simulink model "cartpole_baseline"  (R2026a)
settings: Solver=VariableStepAuto  StopTime=120
InitFcn:
  | cartpole_system_init
undefined symbols (not defined in the file): A, B_u, C, K, L, p, X, x0_i, x0_phys, Y, Z
libraries: sm_lib x9, nesl_utility x3
settings Model: Creator=david  LastModifiedBy=david
settings ExplorerConfigSet: InternalSimMechanicsExplorerSettings=|
  | <ExplorerConfiguration>
  | 
  |   <canonicalview>default</canonicalview>
  | 
  |   <TilePanel>
  |     <TileInfo>
  |       <Tiles Columns="1" Count="1" Height="610" Rows="1" Width="1536">
  |         <Row Weight="1"/>
  |         <Column Weight="1"/>
  |         <Tile Height="1" Width="1" X="0" Y="0"/>
  |       </Tiles>
  |     </TileInfo>
  |     <SceneInfo>
  |       <SceneViewer>
  |         <IsThisViewStd>
  |           <IsStandardView>off</IsStandardView>
  |           <StandardViewName>Front</StandardViewName>
  |         </IsThisViewStd>
  |         <BGColor>
  |           <R>1</R>
  |           <G>1</G>
  |           <B>1</B>
  |           <A>1</A>
  |         </BGColor>
  |         <Camera>
  |           <DoPerspective>off</DoPerspective>
  |           <Position>
  |             <X>-0.38733030516761002</X>
  |             <Y>0.60926147831297028</Y>
  |             <Z>3.3549500429517707</Z>
  |           </Position>
  |           <Center>
  |             <X>-0.38733030516761002</X>
  |             <Y>0.60926147831297028</Y>
  |             <Z>-0.019999999403953556</Z>
  |           </Center>
  |           <Up>
  |             <X>0</X>
  |             <Y>1</Y>
  |             <Z>0</Z>
  |           </Up>
  |           <XLim>1.3855356409800417</XLim>
  |           <YLim>1.3855356409800417</YLim>
  |           <ViewLimDist>0.01</ViewLimDist>
  |         </Camera>
  |       </SceneViewer>
  |     </SceneInfo>
  |   </TilePanel>
  | 
  |   <MechEditorPanel>
  |     <GfxPanelCameraMap/>
  |     <Cameras/>
  |     <VideoCreator>
  |       <IncludeTiles>All</IncludeTiles>
  |       <IncludeTime>on</IncludeTime>
  |       <IncludeWorldFrame>off</IncludeWorldFrame>
  |       <PlaybackSpeedRatio>1</PlaybackSpeedRatio>
  |       <FrameRate>30</FrameRate>
  |       <FrameSize>auto</FrameSize>
  |       <VideoFormat>UncompressedAVI</VideoFormat>
  |     </VideoCreator>
  |   </MechEditorPanel>
  | 
  |   <PlaybackSettings>
  |     <PlaybackSpeedFactor>8</PlaybackSpeedFactor>
  |   </PlaybackSettings>
  | 
  | </ExplorerConfiguration>

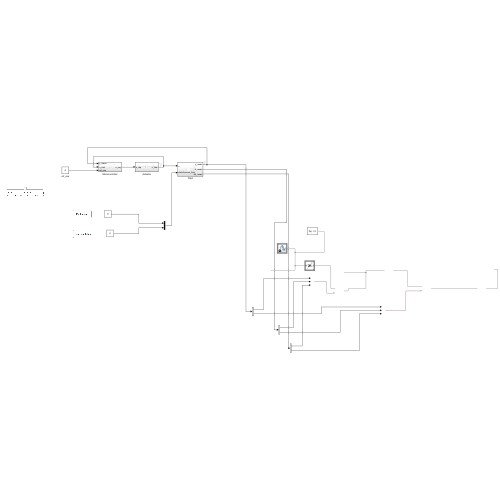
[thumbnail: Simulink's stored preview of the top-level diagram]
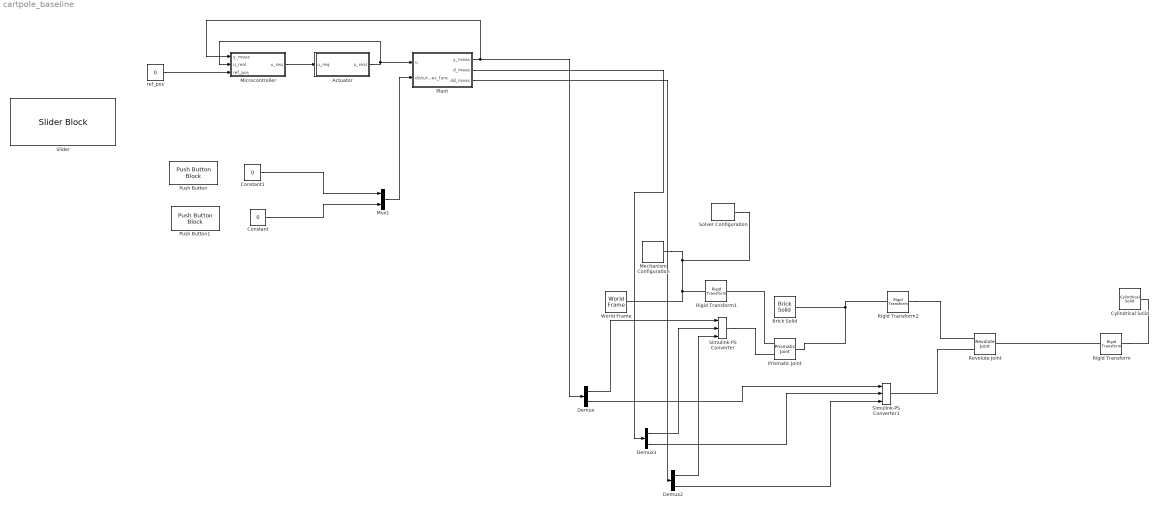
== system cartpole_baseline ==
  Actuator : Subsystem
  Brick Solid : sm_lib/Body Elements/Brick Solid  BrickDimensions=[0.1, 0.15, 0.3]  BrickDimensionsUnits=m  ExportEntireGeometry=off  InertiaType=CalculateFromGeometry  BasedOnType=Mass  Density=1000  DensityUnits=kg/m^3  Mass=p.M  MassUnits=kg  CenterOfMass=[0 0 0]  CenterOfMassUnits=m  MomentsOfInertia=[1 1 1]  MomentsOfInertiaUnits=kg*m^2  ProductsOfInertia=[0 0 0]  ProductsOfInertiaUnits=kg*m^2  GraphicType=FromGeometry  MarkerShape=Sphere  MarkerSize=10  GraphicVisPropType=SimpleVisualProperties  GraphicDiffuseColor=[0.5 0.5 0.5]  GraphicOpacity=1  GraphicSpecularColor=[0.5 0.5 0.5 1.0]  GraphicAmbientColor=[0.15 0.15 0.15 1.0]  GraphicEmissiveColor=[0.0 0.0 0.0 1.0]  GraphicShininess=75  DoExposeReferenceFrame=on  SerializedFrames=<Frames/>
  Constant : Constant  Value=0
  Constant1 : Constant  Value=0
  Cylindrical Solid : sm_lib/Body Elements/Cylindrical Solid  CylinderRadius=0.02  CylinderRadiusUnits=m  CylinderLength=2*p.l  CylinderLengthUnits=m  ExportEntireGeometry=off  InertiaType=CalculateFromGeometry  BasedOnType=Mass  Density=1000  DensityUnits=kg/m^3  Mass=p.m  MassUnits=kg  CenterOfMass=[0 0 0]  CenterOfMassUnits=m  MomentsOfInertia=[1 1 1]  MomentsOfInertiaUnits=kg*m^2  ProductsOfInertia=[0 0 0]  ProductsOfInertiaUnits=kg*m^2  GraphicType=FromGeometry  MarkerShape=Sphere  MarkerSize=10  GraphicVisPropType=SimpleVisualProperties  GraphicDiffuseColor=[0.5 0.5 0.5]  GraphicOpacity=1  GraphicSpecularColor=[0.5 0.5 0.5 1.0]  GraphicAmbientColor=[0.15 0.15 0.15 1.0]  GraphicEmissiveColor=[0.0 0.0 0.0 1.0]  GraphicShininess=75  DoExposeReferenceFrame=on  SerializedFrames=<Frames/>
  Demux : Demux  Outputs=2
  Demux1 : Demux  Outputs=2
  Demux2 : Demux  Outputs=2
  Mechanism Configuration : sm_lib/Utilities/Mechanism Configuration  UniformGravity=Constant  GravityVector=[0 -9.80665 0]  GravityVectorUnits=m/s^2  LinearizationDelta=0.001  JointModeTransitionNonlinearIterations=2
  Microcontroller : Subsystem
  Mux1 : Mux  Inputs=2
  Plant : Subsystem
  Prismatic Joint : sm_lib/Joints/Prismatic Joint  JointMode=Normal  CompositeWrenchDir=FollowerOnBase  CompositeWrenchFrame=BaseFrame  SenseConstraintForce=off  SenseConstraintTorque=off  SenseTotalForce=off  SenseTotalTorque=off  PositionTargetSpecify=off  PositionTargetPriority=High  PositionTargetValue=0  PositionTargetValueUnits=m  VelocityTargetSpecify=off  VelocityTargetPriority=High  VelocityTargetValue=0  VelocityTargetValueUnits=m/s  EquilibriumPosition=0  EquilibriumPositionUnits=m  SpringStiffness=0  SpringStiffnessUnits=N/m  DampingCoefficient=0  DampingCoefficientUnits=N/(m/s)  LowerLimitSpecify=off  LowerLimitBound=-1  LowerLimitBoundUnits=m  LowerLimitStiffness=1e6  LowerLimitStiffnessUnits=N/m  LowerLimitDamping=1e3  LowerLimitDampingUnits=N/(m/s)  LowerLimitTransitionRegionWidth=1e-4  LowerLimitTransitionRegionWidthUnits=m  UpperLimitSpecify=off  UpperLimitBound=1  UpperLimitBoundUnits=m  UpperLimitStiffness=1e6  UpperLimitStiffnessUnits=N/m  UpperLimitDamping=1e3  UpperLimitDampingUnits=N/(m/s)  UpperLimitTransitionRegionWidth=1e-4  UpperLimitTransitionRegionWidthUnits=m  TorqueActuationMode=ComputedTorque  MotionActuationMode=InputMotion  SensePosition=off  SenseVelocity=off  SenseAcceleration=off  SenseTorqueForce=off  SenseLowerLimitTorqueForce=off  SenseUpperLimitTorqueForce=off
  Push Button : PushButtonBlock  ButtonText=Push carrel  OnValue=20  IconOnColor=[0.0, 0.39215686274509803, 0.0]  IconOffColor=[0.0, 1.0, 0.0]  OffValue=0.000000
  Push Button1 : PushButtonBlock  ButtonText=Push pendulum  OnValue=2  IconOnColor=[0.0, 0.39215686274509803, 0.0]  IconOffColor=[0.0, 1.0, 0.0]  OffValue=0.000000
  Revolute Joint : sm_lib/Joints/Revolute Joint  JointMode=Normal  CompositeWrenchDir=FollowerOnBase  CompositeWrenchFrame=BaseFrame  SenseConstraintForce=off  SenseConstraintTorque=off  SenseTotalForce=off  SenseTotalTorque=off  PositionTargetSpecify=off  PositionTargetPriority=High  PositionTargetValue=0  PositionTargetValueUnits=deg  VelocityTargetSpecify=off  VelocityTargetPriority=High  VelocityTargetValue=0  VelocityTargetValueUnits=deg/s  EquilibriumPosition=0  EquilibriumPositionUnits=deg  SpringStiffness=0  SpringStiffnessUnits=N*m/deg  DampingCoefficient=0  DampingCoefficientUnits=N*m/(deg/s)  LowerLimitSpecify=off  LowerLimitBound=-90  LowerLimitBoundUnits=deg  LowerLimitStiffness=1e4  LowerLimitStiffnessUnits=N*m/deg  LowerLimitDamping=10  LowerLimitDampingUnits=N*m/(deg/s)  LowerLimitTransitionRegionWidth=0.1  LowerLimitTransitionRegionWidthUnits=deg  UpperLimitSpecify=off  UpperLimitBound=90  UpperLimitBoundUnits=deg  UpperLimitStiffness=1e4  UpperLimitStiffnessUnits=N*m/deg  UpperLimitDamping=10  UpperLimitDampingUnits=N*m/(deg/s)  UpperLimitTransitionRegionWidth=0.1  UpperLimitTransitionRegionWidthUnits=deg  TorqueActuationMode=ComputedTorque  MotionActuationMode=InputMotion  SensePosition=off  SenseVelocity=off  SenseAcceleration=off  SenseTorqueForce=off  SenseLowerLimitTorqueForce=off  SenseUpperLimitTorqueForce=off
  Rigid Transform : sm_lib/Frames and Transforms/Rigid Transform  RotationMethod=StandardAxis  FollAlignAxisA=+X  BaseAlignAxisA=+Y  FollAlignAxisB=+Y  BaseAlignAxisB=+Z  RotationStandardAxis=+X  RotationAngle=90  RotationAngleUnits=deg  RotationArbitraryAxis=[0 0 1]  RotationSequenceAxes=FollowerAxes  RotationSequence=XYX  RotationSequenceAngles=[0 0 0]  RotationSequenceAnglesUnits=deg  RotationMatrix=[1 0 0;0 1 0;0 0 1]  Quaternion=[1 0 0 0]  TranslationMethod=Cartesian  TranslationCartesianOffset=[0 p.l 0]  TranslationCartesianOffsetUnits=m  TranslationStandardAxis=+Z  TranslationStandardOffset=p.l  TranslationStandardOffsetUnits=m  TranslationROffset=0  TranslationROffsetUnits=m  TranslationThetaOffset=0  TranslationThetaOffsetUnits=deg  TranslationZOffset=0  TranslationZOffsetUnits=m
  Rigid Transform1 : sm_lib/Frames and Transforms/Rigid Transform  RotationMethod=StandardAxis  FollAlignAxisA=+X  BaseAlignAxisA=+Y  FollAlignAxisB=+Y  BaseAlignAxisB=+Z  RotationStandardAxis=+Y  RotationAngle=90  RotationAngleUnits=deg  RotationArbitraryAxis=[0 0 1]  RotationSequenceAxes=FollowerAxes  RotationSequence=XYX  RotationSequenceAngles=[0 0 0]  RotationSequenceAnglesUnits=deg  RotationMatrix=[1 0 0;0 1 0;0 0 1]  Quaternion=[1 0 0 0]  TranslationMethod=None  TranslationCartesianOffset=[0 0 0]  TranslationCartesianOffsetUnits=m  TranslationStandardAxis=+Z  TranslationStandardOffset=0  TranslationStandardOffsetUnits=m  TranslationROffset=0  TranslationROffsetUnits=m  TranslationThetaOffset=0  TranslationThetaOffsetUnits=deg  TranslationZOffset=0  TranslationZOffsetUnits=m
  Rigid Transform2 : sm_lib/Frames and Transforms/Rigid Transform  RotationMethod=StandardAxis  FollAlignAxisA=+X  BaseAlignAxisA=+Y  FollAlignAxisB=+Y  BaseAlignAxisB=+Z  RotationStandardAxis=+Y  RotationAngle=90  RotationAngleUnits=deg  RotationArbitraryAxis=[0 0 1]  RotationSequenceAxes=FollowerAxes  RotationSequence=XYX  RotationSequenceAngles=[0 0 0]  RotationSequenceAnglesUnits=deg  RotationMatrix=[1 0 0;0 1 0;0 0 1]  Quaternion=[1 0 0 0]  TranslationMethod=Cartesian  TranslationCartesianOffset=[0.07, 0, 0]  TranslationCartesianOffsetUnits=m  TranslationStandardAxis=+Z  TranslationStandardOffset=0  TranslationStandardOffsetUnits=m  TranslationROffset=0  TranslationROffsetUnits=m  TranslationThetaOffset=0  TranslationThetaOffsetUnits=deg  TranslationZOffset=0  TranslationZOffsetUnits=m
  Simulink-PS Converter : nesl_utility/Simulink-PS Converter  PhysicalDomain=network_engine_domain  SubClassName=ps_input  LeftPortType=input  RightPortType=output  PseudoPeriodic=off  Frequencies=[]  NoiseDistribution=none  NoiseParameters=[]  Unit=1  AffineConversion=off  FilteringAndDerivatives=provide  SimscapeFilterOrder=2  InputFilterTimeConstant=0.001  UdotUserProvided=2
  Simulink-PS Converter1 : nesl_utility/Simulink-PS Converter  PhysicalDomain=network_engine_domain  SubClassName=ps_input  LeftPortType=input  RightPortType=output  PseudoPeriodic=off  Frequencies=[]  NoiseDistribution=none  NoiseParameters=[]  Unit=1  AffineConversion=on  FilteringAndDerivatives=provide  SimscapeFilterOrder=2  InputFilterTimeConstant=0.001  UdotUserProvided=2
  Slider : SliderBlock  LabelPosition=Hide  ScaleMin=-1  ScaleMax=1
  Solver Configuration : nesl_utility/Solver Configuration  PhysicalDomain=network_engine_domain  SubClassName=solver  LeftPortType=input  RightPortType=generic  Tones=[]  Harmonics=[]  SimulateNoise=off  Profile=off  UseLocalSampling=off  EnableSwitchedLinearOptims=on  FrequencyDomain=off  UseCCode=off  RelTol=0.001  AbsTol=0.001  MinStep=1e-09  ToWorkspace=off  RevertToSquareIcSolve=off  NumHomotopyIterations=100  PhasorMode=off  PhasorModeNumHarmonics=1  ConsistencySolver=NEWTON_XTOL_AFTER_FTOL  CanonicalOrdering=CANONICAL  OptimizeIntermediates=OPTIMIZED  IndexReductionMethod=DerivativeReplacement  DoDC=off  ResidualTolerance=1e-09  ConsistencyTolSource=GLOBAL  ConsistencyAbsTol=0.001  ConsistencyRelTol=0.001  ConsistencyTolFactor=0.001  UseLocalSolver=off  LocalSolverChoice=NE_BACKWARD_EULER_ADVANCER  ResolveIndetEquations=on  FunctionEvalNumThread=1  LocalSolverSampleTime=0.001  DoFixedCost=off  MaxNonlinIter=3  MaxModeIter=2  ComputeImpulses=off  ImpulseIterations=2  LinearAlgebra=auto  LinearAlgebraNumThread=0  EquationFormulation=NE_TIME_EF  DelaysMemoryBudget=1024  AutomaticFiltering=on  FilteringTimeConstant=0.001  PartitionStorageMethod=AS_NEEDED  PartitionMemoryBudget=1024  PartitionMethod=ROBUST  MultibodyUseLocalSolver=off  MultibodyLocalSolverChoice=ODE1  MultibodyLocalSolverSampleTime=0.001
  World Frame : sm_lib/Frames and Transforms/World Frame
  ref_pos : Constant  Value=0
  wires:
  Demux2/1 -> Simulink-PS Converter/3
  Demux2/2 -> Simulink-PS Converter1/3
  Plant/1(y_meas) -> Microcontroller/1(y_meas), Demux/1
  Microcontroller/1(u_req) -> Actuator/1(u_req)
  Plant/2(d_meas) -> Demux1/1
  Actuator/1(u_real) -> Microcontroller/2(u_real), Plant/1(u)
  Plant/3(dd_meas) -> Demux2/1
  Demux/1 -> Simulink-PS Converter/1
  Demux1/2 -> Simulink-PS Converter1/2
  Demux1/1 -> Simulink-PS Converter/2
  Demux/2 -> Simulink-PS Converter1/1
  Constant1/1 -> Mux1/1
  Constant/1 -> Mux1/2
  Mux1/1 -> Plant/2(disturbances_func)
  ref_pos/1 -> Microcontroller/3(ref_pos)
  connections:
  Brick Solid/RConn1 -- Prismatic Joint/RConn1 -- Rigid Transform2/LConn1
  Mechanism Configuration/RConn1 -- World Frame/RConn1 -- Rigid Transform1/LConn1 -- Solver Configuration/RConn1
  Rigid Transform2/RConn1 -- Revolute Joint/LConn1
  Simulink-PS Converter/RConn1 -- Prismatic Joint/LConn2
  Rigid Transform/RConn1 -- Cylindrical Solid/RConn1
  Revolute Joint/LConn2 -- Simulink-PS Converter1/RConn1
  Rigid Transform/LConn1 -- Revolute Joint/RConn1
  Prismatic Joint/LConn1 -- Rigid Transform1/RConn1

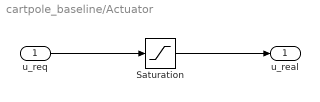
== system cartpole_baseline/Actuator ==
  u_req : Inport
  Saturation : Saturate  UpperLimit=p.U_MAX  LowerLimit=-p.U_MAX
  u_real : Outport
  wires:
  u_req/1 -> Saturation/1
  Saturation/1 -> u_real/1

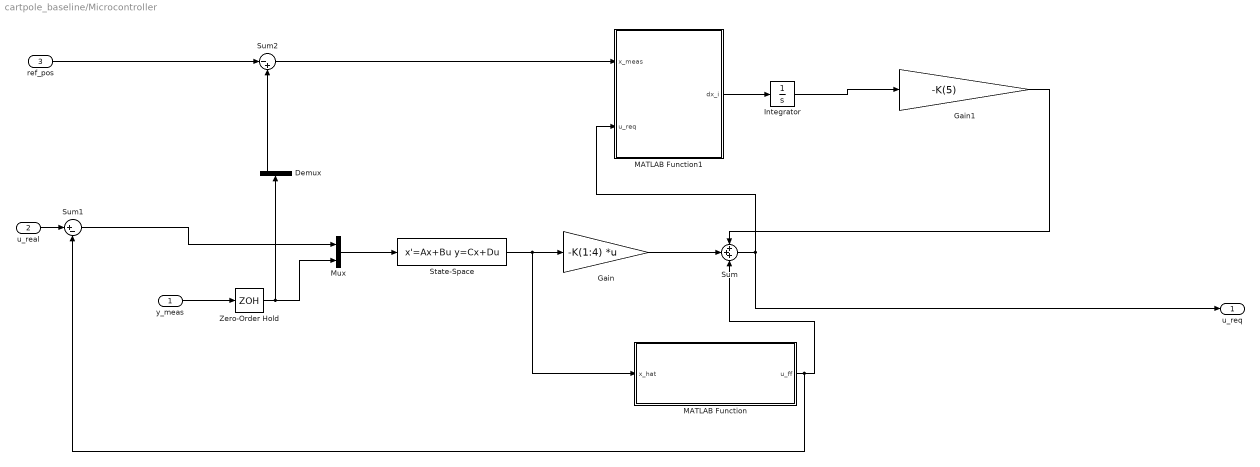
== system cartpole_baseline/Microcontroller ==
  y_meas : Inport
  u_real : Inport  Port=2
  ref_pos : Inport  Port=3
  Demux : Demux  Outputs=2
  Gain : Gain  Gain=-K(1:4)  Multiplication=Matrix(K*u)
  Gain1 : Gain  Gain=-K(5)
  Integrator : Integrator  InitialCondition=x0_i
  MATLAB Function : MATLAB Function  TreatAsAtomicUnit=on
  MATLAB Function1 : MATLAB Function  TreatAsAtomicUnit=on
  Mux : Mux  Inputs=[1, 2]
  State-Space : StateSpace  A=A-L*C  B=[B_u, L]  C=eye(4)  D=zeros(4, 3)  InitialCondition=x0_phys
  Sum : Sum  Inputs=+++
  Sum1 : Sum  Inputs=|+-
  Sum2 : Sum  Inputs=|-+
  Zero-Order Hold : ZeroOrderHold  SampleTime=0.01
  u_req : Outport
  wires:
  y_meas/1 -> Zero-Order Hold/1
  State-Space/1 -> MATLAB Function/1(x_hat), Gain/1
  Mux/1 -> State-Space/1
  Sum/1 -> u_req/1, MATLAB Function1/2(u_req)
  MATLAB Function1/1(dx_i) -> Integrator/1
  Gain/1 -> Sum/2
  MATLAB Function/1(u_ff) -> Sum/3, Sum1/2
  Integrator/1 -> Gain1/1
  Gain1/1 -> Sum/1
  u_real/1 -> Sum1/1
  Sum1/1 -> Mux/1
  Zero-Order Hold/1 -> Mux/2, Demux/1
  ref_pos/1 -> Sum2/1
  Demux/1 -> Sum2/2
  Sum2/1 -> MATLAB Function1/1(x_meas)

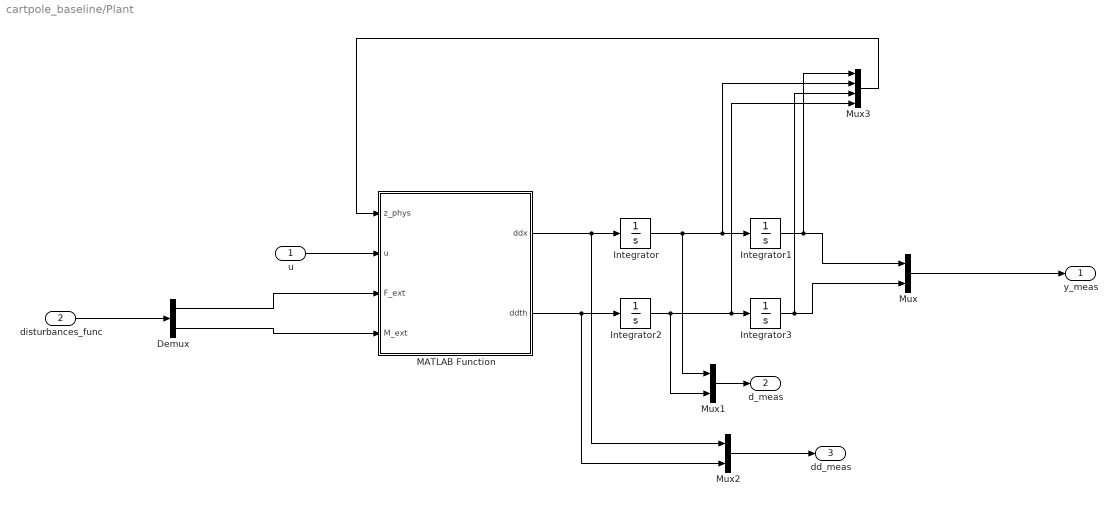
== system cartpole_baseline/Plant ==
  u : Inport
  disturbances_func : Inport  Port=2
  Demux : Demux  Outputs=2
  Integrator : Integrator  InitialCondition=x0_phys(2)
  Integrator1 : Integrator  InitialCondition=x0_phys(1)
  Integrator2 : Integrator  InitialCondition=x0_phys(4)
  Integrator3 : Integrator  InitialCondition=x0_phys(3)
  MATLAB Function : MATLAB Function  TreatAsAtomicUnit=on
  Mux : Mux  Inputs=2
  Mux1 : Mux  Inputs=2
  Mux2 : Mux  Inputs=2
  Mux3 : Mux
  y_meas : Outport
  d_meas : Outport  Port=2
  dd_meas : Outport  Port=3
  wires:
  MATLAB Function/1(ddx) -> Integrator/1, Mux2/1
  MATLAB Function/2(ddth) -> Integrator2/1, Mux2/2
  Integrator2/1 -> Mux3/4, Integrator3/1, Mux1/2
  Integrator/1 -> Mux3/2, Integrator1/1, Mux1/1
  u/1 -> MATLAB Function/2(u)
  Integrator1/1 -> Mux/1, Mux3/1
  Integrator3/1 -> Mux3/3, Mux/2
  Mux/1 -> y_meas/1
  Mux1/1 -> d_meas/1
  Mux2/1 -> dd_meas/1
  disturbances_func/1 -> Demux/1
  Demux/1 -> MATLAB Function/3(F_ext)
  Demux/2 -> MATLAB Function/4(M_ext)
  Mux3/1 -> MATLAB Function/1(z_phys)

== matlab function cartpole_baseline/Microcontroller/MATLAB Function ==
  data: x_hat input; u_ff output; p parameter
function u_ff = friction_feedforward(x_hat, p)
    th_hat  = x_hat(3);
    dth_hat = x_hat(4);
    dx_hat  = x_hat(2);
    
    N_approx_est  = max(0, (-p.beta_m*sin(th_hat)*dth_hat + p.l*(p.M*p.g + p.m*(p.g*cos(th_hat) - p.l*dth_hat^2)*cos(th_hat)))/p.l);
    F_coulomb_est = p.mu_c * N_approx_est;
    u_ff = p.ff_compensation * F_coulomb_est * tanh(p.k * x_hat(2));
end

== matlab function cartpole_baseline/Plant/MATLAB Function ==
  data: z_phys input; u input; p parameter; F_ext input; M_ext input; ddx output; ddth output
function [ddx, ddth] = system_dynamics(z_phys, u, p, F_ext, M_ext)

    % z_phys = [x; dx; th; dth]
    dx  = z_phys(2);
    th  = z_phys(3);
    dth = z_phys(4);

    N_approx_real = max(0, (-dth.*p.beta_m.*sin(th) + p.l.*(p.M.*p.g + p.m.*(-dth.^2.*p.l + p.g.*cos(th)).*cos(th)))./p.l);
    M_mat = [p.M + p.m.*sin(th).^2 0; p.m.*cos(th) p.l.*p.m];
    F_vec = [F_ext - N_approx_real.*(p.mu_c + (-p.mu_c + p.mu_s).*exp(-dx.^2./p.v_s.^2)).*tanh(dx.*p.k) + dth.*p.beta_m.*cos(th)./p.l - dx.*p.beta_M + p.m.*(dth.^2.*p.l - p.g.*cos(th)).*sin(th) + u; M_ext./p.l - dth.*p.beta_m./p.l + p.g.*p.m.*sin(th)];

    q_ddot = M_mat \ F_vec;

    ddx  = q_ddot(1);
    ddth = q_ddot(2);

end

== matlab function cartpole_baseline/Microcontroller/MATLAB Function1 ==
  data: x_meas input; dx_i output; u_req input; p parameter
function dx_i = anti_windup_logic(x_meas, u_req, p)
    dx_i = x_meas;
    
    if (u_req >= p.U_MAX && dx_i > 0) || (u_req <= -p.U_MAX && dx_i < 0)
        dx_i = 0;
    end
end
